simulink model "exp1_latest_work_of_FULL_HEART_PICTURE_orignal_pure"  (R2023a)
settings: Solver=VariableStepAuto  StartTime=0.0  StopTime=60  RelTol=1e-3  AbsTol=1e-3
libraries: fl_lib x38, sh_lib x21, nesl_utility x19, simulink x7, Cardiovascular_lib x4
(part 2 of 2)

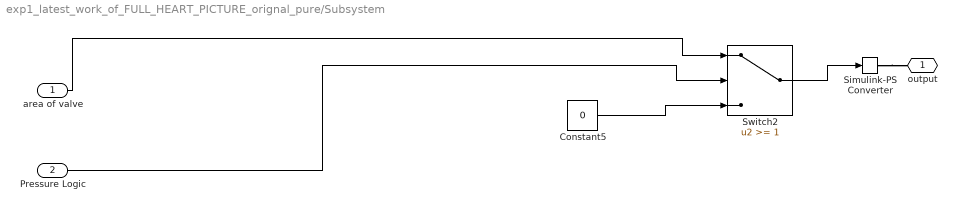
== system exp1_latest_work_of_FULL_HEART_PICTURE_orignal_pure/Subsystem ==
  area of valve : Inport
  "Pressure Logic " : Inport  Port=2
  Constant5 : Constant  Value=0
  Simulink-PS Converter : nesl_utility/Simulink-PS Converter  PhysicalDomain=network_engine_domain  SubClassName=ps_input  LeftPortType=input  RightPortType=output  PseudoPeriodic=off  Frequencies=[]  NoiseDistribution=none  NoiseParameters=[]  Unit=1  AffineConversion=off  FilteringAndDerivatives=provide  SimscapeFilterOrder=1  InputFilterTimeConstant=0.001  UdotUserProvided=0
  Switch2 : Switch  Threshold=1  SaturateOnIntegerOverflow=off  InputSameDT=off
  output : PMIOPort  Side=Left
  wires:
  area of valve/1 -> Switch2/1
  Constant5/1 -> Switch2/3
  Switch2/1 -> Simulink-PS Converter/1
  "Pressure Logic "/1 -> Switch2/2
  connections:
  Simulink-PS Converter/RConn1 -- output/RConn1

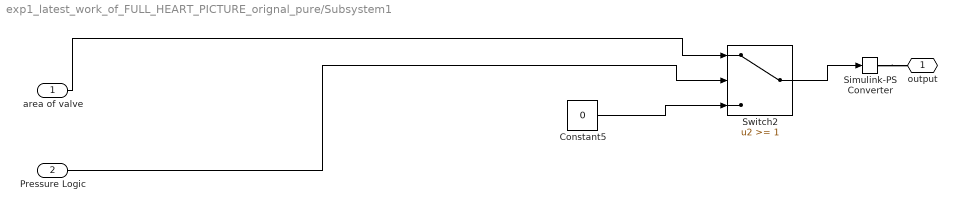
== system exp1_latest_work_of_FULL_HEART_PICTURE_orignal_pure/Subsystem1 ==
  area of valve : Inport
  "Pressure Logic " : Inport  Port=2
  Constant5 : Constant  Value=0
  Simulink-PS Converter : nesl_utility/Simulink-PS Converter  PhysicalDomain=network_engine_domain  SubClassName=ps_input  LeftPortType=input  RightPortType=output  PseudoPeriodic=off  Frequencies=[]  NoiseDistribution=none  NoiseParameters=[]  Unit=1  AffineConversion=off  FilteringAndDerivatives=provide  SimscapeFilterOrder=1  InputFilterTimeConstant=0.001  UdotUserProvided=0
  Switch2 : Switch  Threshold=1  SaturateOnIntegerOverflow=off  InputSameDT=off
  output : PMIOPort  Side=Left
  wires:
  area of valve/1 -> Switch2/1
  Constant5/1 -> Switch2/3
  Switch2/1 -> Simulink-PS Converter/1
  "Pressure Logic "/1 -> Switch2/2
  connections:
  Simulink-PS Converter/RConn1 -- output/RConn1

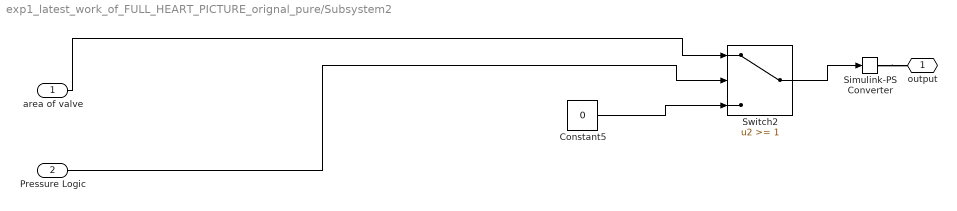
== system exp1_latest_work_of_FULL_HEART_PICTURE_orignal_pure/Subsystem2 ==
  area of valve : Inport
  "Pressure Logic " : Inport  Port=2
  Constant5 : Constant  Value=0
  Simulink-PS Converter : nesl_utility/Simulink-PS Converter  PhysicalDomain=network_engine_domain  SubClassName=ps_input  LeftPortType=input  RightPortType=output  PseudoPeriodic=off  Frequencies=[]  NoiseDistribution=none  NoiseParameters=[]  Unit=1  AffineConversion=off  FilteringAndDerivatives=provide  SimscapeFilterOrder=1  InputFilterTimeConstant=0.001  UdotUserProvided=0
  Switch2 : Switch  Threshold=1  SaturateOnIntegerOverflow=off  InputSameDT=off
  output : PMIOPort  Side=Left
  wires:
  area of valve/1 -> Switch2/1
  Constant5/1 -> Switch2/3
  Switch2/1 -> Simulink-PS Converter/1
  "Pressure Logic "/1 -> Switch2/2
  connections:
  Simulink-PS Converter/RConn1 -- output/RConn1

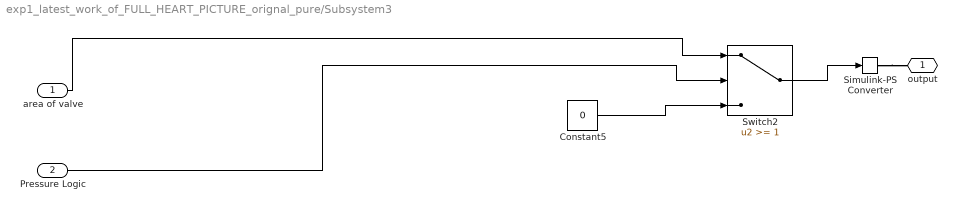
== system exp1_latest_work_of_FULL_HEART_PICTURE_orignal_pure/Subsystem3 ==
  area of valve : Inport
  "Pressure Logic " : Inport  Port=2
  Constant5 : Constant  Value=0
  Simulink-PS Converter : nesl_utility/Simulink-PS Converter  PhysicalDomain=network_engine_domain  SubClassName=ps_input  LeftPortType=input  RightPortType=output  PseudoPeriodic=off  Frequencies=[]  NoiseDistribution=none  NoiseParameters=[]  Unit=1  AffineConversion=off  FilteringAndDerivatives=provide  SimscapeFilterOrder=1  InputFilterTimeConstant=0.001  UdotUserProvided=0
  Switch2 : Switch  Threshold=1  SaturateOnIntegerOverflow=off  InputSameDT=off
  output : PMIOPort  Side=Left
  wires:
  area of valve/1 -> Switch2/1
  Constant5/1 -> Switch2/3
  Switch2/1 -> Simulink-PS Converter/1
  "Pressure Logic "/1 -> Switch2/2
  connections:
  Simulink-PS Converter/RConn1 -- output/RConn1

== stateflow chart exp1_latest_work_of_FULL_HEART_PICTURE_orignal_pure/mitral valve ==
  state off
    en:y=0;
  state on
    en:y=1;
  (default) -> off
  on -> off : [x<200]
  off -> on : [x>600]
  data: x input; y output

== stateflow chart exp1_latest_work_of_FULL_HEART_PICTURE_orignal_pure/aortic valve ==
  state off
    en:y=0;
  state on
    en:y=1;
  (default) -> off
  on -> off : [x<4000]
  off -> on : [x>9000]
  data: x input; y output

== stateflow chart exp1_latest_work_of_FULL_HEART_PICTURE_orignal_pure/pulmonary valve1 ==
  state off
    en:y=0;
  state on
    en:y=1;
  (default) -> off
  on -> off : [x<1500]
  off -> on : [x>2000]
  data: x input; y output

== stateflow chart exp1_latest_work_of_FULL_HEART_PICTURE_orignal_pure/pulmonary valve ==
  state off
    en:y=0;
  state on
    en:y=1;
  (default) -> off
  on -> off : [x<1500]
  off -> on : [x>2000]
  data: x input; y output

== matlab function exp1_latest_work_of_FULL_HEART_PICTURE_orignal_pure/MATLAB Function ==
  settings: updateMethod=DISCRETE
  data: u input; y output
function y = moving_average(u)
    % Parameters
    persistent buffer;
    N = 1000; % Number of samples in the moving average window

    if isempty(buffer)
        buffer = zeros(N, 1);
    end

    % Update the buffer
    buffer = [buffer(2:end); u];

    % Compute the moving average
    y = mean(buffer);
end
